simulink model "Trajectory_generation"  (R2021b)
settings: Solver=VariableStepAuto  StartTime=0.0  StopTime=30  RelTol=1e-3
PreLoadFcn:
  | coeffsCA = load(strcat( dataPath, '/CAinterpCoeffs.mat'));
undefined symbols (not defined in the file or in its folder): deltaX, settingsSim, Vx_final, Vy_final, Vz_final, Vz_initial, x_final, y_final, z_final
settings Model: PacingRate=0.350000  Creator=adm-w10  LastModifiedBy=marco
settings SolverCC: AlgebraicLoopSolver=TrustRegion
settings DebuggingCC: SFMachineParentedDataDiag=warning
settings SFSimCC: CustomCodeUndefinedFunction=UseInterfaceOnly

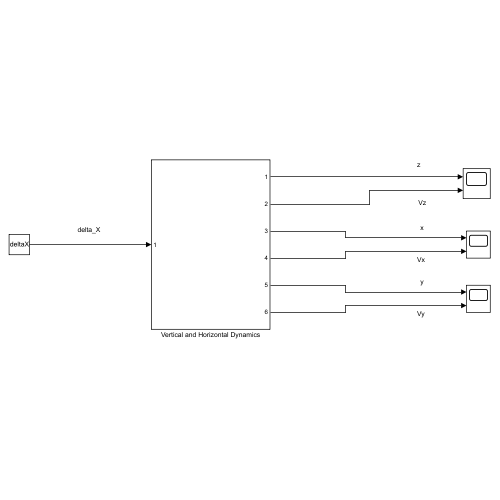
[thumbnail: Simulink's stored preview of the top-level diagram]
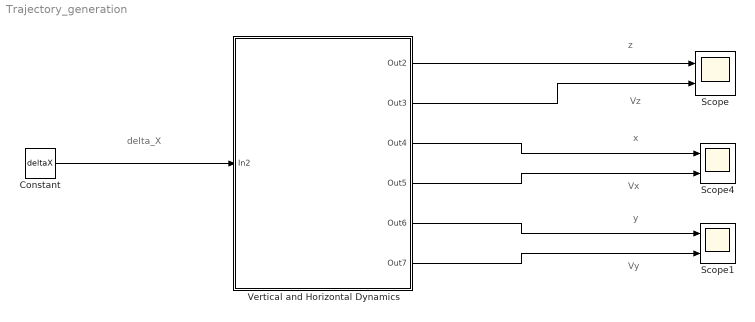
== system Trajectory_generation ==
  note: delta_X
  note: Vz
  note: z
  note: Vx
  note: x
  note: Vy
  note: y
  Constant : Constant  Value=deltaX
  Scope : Scope  NumInputPorts=2
  Scope1 : Scope  NumInputPorts=2
  Scope4 : Scope  NumInputPorts=2
  Vertical and Horizontal Dynamics : Subsystem
  wires:
  Constant/1 -> Vertical and Horizontal Dynamics/1(In2)
  Vertical and Horizontal Dynamics/3(Out4) -> Scope4/1
  Vertical and Horizontal Dynamics/4(Out5) -> Scope4/2
  Vertical and Horizontal Dynamics/1(Out2) -> Scope/1
  Vertical and Horizontal Dynamics/2(Out3) -> Scope/2
  Vertical and Horizontal Dynamics/5(Out6) -> Scope1/1
  Vertical and Horizontal Dynamics/6(Out7) -> Scope1/2

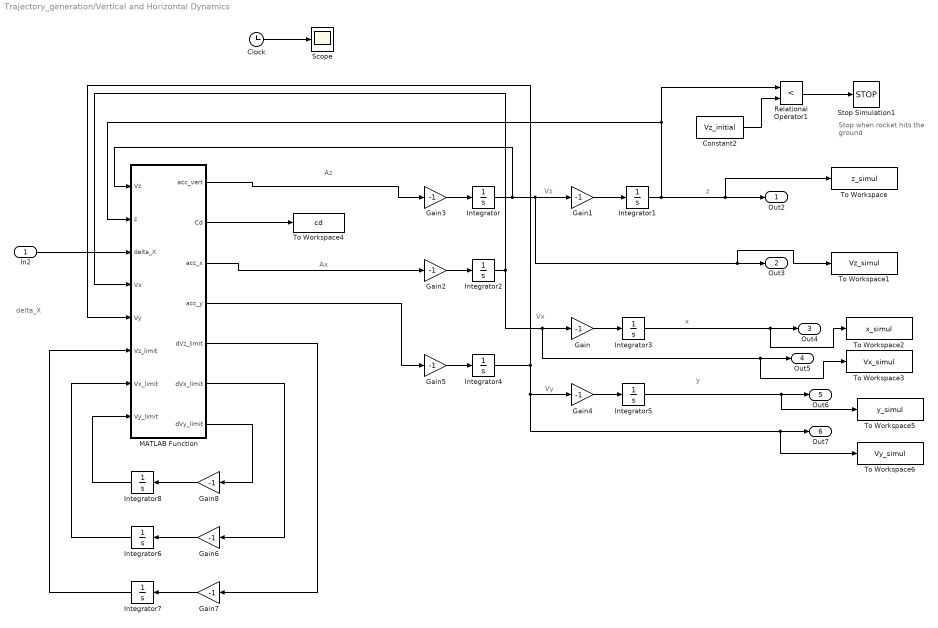
== system Trajectory_generation/Vertical and Horizontal Dynamics ==
  note: delta_X
  note: Az
  note: x
  note: Vz
  note: Stop when rocket
      |  hits the ground
  note: Ax
  note: y
  note: z
  note: Vy
  note: Vx
  In2 : Inport
  Clock : Clock
  Constant2 : Constant  Value=Vz_initial
  Gain{,1..8} (9 alike) : Gain  Gain=-1
  Integrator : Integrator  InitialCondition=Vz_final
  Integrator1 : Integrator  InitialCondition=z_final
  Integrator2 : Integrator  InitialCondition=Vx_final
  Integrator3 : Integrator  InitialCondition=x_final
  Integrator4 : Integrator  InitialCondition=Vy_final
  Integrator5 : Integrator  InitialCondition=y_final
  Integrator6 : Integrator  InitialCondition=Vx_final
  Integrator7 : Integrator  InitialCondition=Vz_final
  Integrator8 : Integrator  InitialCondition=Vy_final
  MATLAB Function : MATLAB Function  TreatAsAtomicUnit=on  SystemSampleTime=0.05
  Relational Operator1 : RelationalOperator  Operator=<  OutDataTypeStr=boolean  RndMeth=Simplest
  Scope : Scope
  Stop Simulation1 : Stop
  To Workspace : ToWorkspace  VariableName=z_simul  SampleTime=-1
  To Workspace1 : ToWorkspace  VariableName=Vz_simul  SampleTime=-1
  To Workspace2 : ToWorkspace  VariableName=x_simul  SampleTime=-1
  To Workspace3 : ToWorkspace  VariableName=Vx_simul  SampleTime=-1
  To Workspace4 : ToWorkspace  VariableName=cd  SampleTime=-1
  To Workspace5 : ToWorkspace  VariableName=y_simul  SampleTime=-1
  To Workspace6 : ToWorkspace  VariableName=Vy_simul  SampleTime=-1
  Out2 : Outport  VectorParamsAs1DForOutWhenUnconnected=off
  Out3 : Outport  Port=2  VectorParamsAs1DForOutWhenUnconnected=off
  Out4 : Outport  Port=3  VectorParamsAs1DForOutWhenUnconnected=off
  Out5 : Outport  Port=4  VectorParamsAs1DForOutWhenUnconnected=off
  Out6 : Outport  Port=5  VectorParamsAs1DForOutWhenUnconnected=off
  Out7 : Outport  Port=6  VectorParamsAs1DForOutWhenUnconnected=off
  wires:
  Integrator5/1 -> Out6/1, To Workspace5/1
  Integrator4/1 -> Gain4/1, To Workspace6/1, Out7/1, MATLAB Function/5(Vy)
  MATLAB Function/1(acc_vert) -> Gain3/1
  Integrator1/1 -> Relational Operator1/1, MATLAB Function/2(z), Out2/1, To Workspace/1
  In2/1 -> MATLAB Function/3(delta_X)
  Gain5/1 -> Integrator4/1
  Gain2/1 -> Integrator2/1
  Relational Operator1/1 -> Stop Simulation1/1
  MATLAB Function/3(acc_x) -> Gain2/1
  Gain1/1 -> Integrator1/1
  Gain/1 -> Integrator3/1
  Integrator3/1 -> To Workspace2/1, Out4/1
  Gain4/1 -> Integrator5/1
  Gain3/1 -> Integrator/1
  Constant2/1 -> Relational Operator1/2
  Integrator2/1 -> To Workspace3/1, Out5/1, Gain/1, MATLAB Function/4(Vx)
  MATLAB Function/4(acc_y) -> Gain5/1
  Integrator/1 -> MATLAB Function/1(Vz), Gain1/1, Out3/1, To Workspace1/1
  MATLAB Function/2(Cd) -> To Workspace4/1
  Clock/1 -> Scope/1
  MATLAB Function/5(dVz_limit) -> Gain7/1
  MATLAB Function/6(dVx_limit) -> Gain6/1
  Integrator6/1 -> MATLAB Function/7(Vx_limit)
  Integrator7/1 -> MATLAB Function/6(Vz_limit)
  Gain6/1 -> Integrator6/1
  Gain7/1 -> Integrator7/1
  MATLAB Function/7(dVy_limit) -> Gain8/1
  Integrator8/1 -> MATLAB Function/8(Vy_limit)
  Gain8/1 -> Integrator8/1

== matlab function Trajectory_generation/Vertical and Horizontal Dynamics/MATLAB Function ==
  data: Vz input; z input; delta_X input; acc_vert output; Cd output; acc_x output; Vx input; Vy input; acc_y output; coeffsCA parameter; settingsSim parameter; Vz_limit input; Vx_limit input; dVz_limit output; dVx_limit output; Vy_limit input; dVy_limit output
function [acc_vert, Cd, acc_x, acc_y,dVz_limit, dVx_limit,dVy_limit] = model(Vz, z, delta_X, Vx, Vy, coeffsCA, settingsSim,Vz_limit, Vx_limit,Vy_limit)
%{ 

model - ode model to compute a back integration of the rocket dynamics

INTPUTS: 
            - Vz
            - Z
            - delta_x
            - Vx
            - Vy
            - coeffsCA     
            - settingsSim
            - Vz_limit
            - Vx_limit
OUTPUTS:
            - Tf, array, Total integration time vector; 
            - Yf, array, Total State Matrix;
            - Ta, array, [n� variations, 1], Ascent Integration time vector;
            - Ya, array, [n� variations, 16], Ascent State Matrix;
            - bound_value, struct, Useful values for the plots;

CALLED FUNCTIONS: windConstGenerator, ascent, recallOdeFcn, descentParachute, descentParachute6Dof, delayControl.

REVISIONS:
- 0                 Release, Ruben Di Battista
- 1                 Revision, Francesco Colombi
- 2     09/10/2019, Revision, Adriano Filippo Inno
- 3     16/04/2021, Update,   Fiammetta Artioli, Davide Rosato
                    6DOF descent update
- 4     03/10/2021, Update,   Davide Rosato
                    Multiple smooth airbrakes opening update
Copyright © 2021, Skyward Experimental Rocketry, AFD department
All rights reserved

SPDX-License-Identifier: GPL-3.0-or-later

%}


% Parameters
ro         = getRho(z + settingsSim.z0);
m          = settingsSim.ms;
g          = settingsSim.g0;
diameter   = settingsSim.C; 
S0         = (pi*diameter^2)/4; 


% Compute the modulus of velocity
V_mod = sqrt(Vx^2 + Vz^2 + Vy^2);

% Obtain the Cd value ( It includes also the airbrake surface )
Cd = getDrag(V_mod, z + settingsSim.z0, delta_X, coeffsCA.coeffs);

% Compute the vertical and horizontal accelerations using the dynamic equations
acc_vert  = (-0.5*ro*S0*Cd*Vz*V_mod - m*g)/m;
acc_x     = (-0.5*ro*S0*Cd*Vx*V_mod)/m;
acc_y     = (-0.5*ro*S0*Cd*Vy*V_mod)/m;

V_mod_limit = 350; 
% this is to avoid having speed going to infinity:
% approaching the ground as the backintegration continues to increase the
% forces acting on the rocket, the trajectories generated have the tendancy
% to diverge to infinite speed, but this is something not physical

if V_mod <= V_mod_limit
    dVz_limit = acc_vert;
    dVx_limit = acc_x;
    dVy_limit = acc_y;
else
    dVz_limit = 0;
    dVx_limit = 0;
    dVy_limit = 0;
    Cd = getDrag(V_mod_limit, z + settingsSim.z0, delta_X, coeffsCA.coeffs);
end

if V_mod > V_mod_limit
    acc_vert  = (-0.5*ro*S0*Cd*Vz_limit*V_mod_limit - m*g)/m;
    acc_x     = (-0.5*ro*S0*Cd*Vx_limit*V_mod_limit)/m;
    acc_y     = (-0.5*ro*S0*Cd*Vy_limit*V_mod_limit)/m;
end
